simulink model "example1"  (Simulink 10.1)
settings: Solver=ode45  StartTime=0.0  StopTime=15  FixedStep=1e-2  MaxStep=1e-2  RelTol=1e-3  EnableMultiTasking=on
libraries: simulink x3
settings Model: Creator=marcelo  LastModifiedBy=maxwe
settings SolverCC: ZeroCrossAlgorithm=Non-adaptive
settings DataIOCC: SignalLoggingSaveFormat=ModelDataLogs  SaveOutput=off
settings OptimizationCC: ExpressionDepthLimit=2147483647  InitFltsAndDblsToZero=on
settings DebuggingCC: SaveWithParameterizedLinksMsg=none  SignalResolutionControl=TryResolveAllWithWarning  SolverPrmCheckMsg=warning  MultiTaskDSMMsg=warning  MultiTaskCondExecSysMsg=none  FcnCallInpInsideContextMsg=warning  StateNameClashWarn=warning
settings SFSimCC: SimUseLocalCustomCode=on  CustomCodeUndefinedFunction=FilterOut
settings RTWCC: RTWUseLocalCustomCode=on
settings GRTTargetCC: TargetFcnLib=ansi_tfl_tmw.mat
settings ConfigComp: CovExternalEMLEnable=on

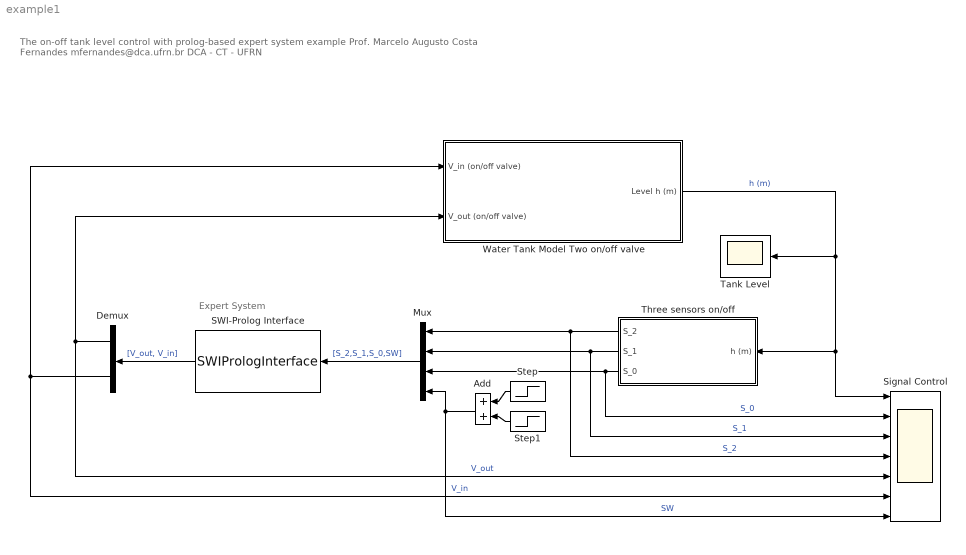
== system example1 ==
  note: Expert System
  note: The on-off tank level control with prolog-based expert system example
      | Prof. Marcelo Augusto Costa Fernandes
      | mfernandes@dca.ufrn.br
      | DCA - CT - UFRN
  Add : Sum
  Demux : Demux  Outputs=2
  Mux : Mux
  SWI-Prolog Interface : S-Function  FunctionName=SWIPrologInterface  Parameters=jplPath, plFile, nIn, plQuery, nOut,0  SFunctionDeploymentMode=off  EnableBusSupport=off  mask(SWI-Prolog (www.swi-prolog.org) Interface){jplPath=E:\Program Files\swipl\lib\jpl.jar, plFile=example1Prolog.pl, nIn=4, nOut=2, plQuery=control(y(2),y(1),u(3),u(2),u(1),u(4))}
      mask prompts: jplPath "Path of the JPL jar-file:"; plFile "Prolog file:"; nIn "Number of the inputs:"; nOut "Number of the outputs:"; plQuery "Prolog query:"
      mask help:
      | SWI-Prolog (www.swi-prolog.org) Interface block.
      |
      | Execute Prolog code (PL file) in the Simulink environment.
      |
      | Use ''u'' as the input variable name and ''y'' as the output variable name.
      |
      | In the case of queries with multiple solutions, this block will only return the first solution found.
      |
      | Prof. Marcelo Augusto Costa Fernandes
      | mfernandes@dca.ufrn.br
      | DCA - CT - UFRN
      mask Help:
      | SWI-Prolog (www.swi-prolog.org) Interface block.
      | 
      | Execute Prolog code (PL file) in the Simulink environment.
      | 
      | Use ''u'' as the input variable name and ''y'' as the output variable name.
      | 
      | In the case of queries with multiple solutions, this block will only return the first solution found.
      | 
      | Prof. Marcelo Augusto Costa Fernandes
      | mfernandes@dca.ufrn.br
      | DCA - CT - UFRN
      mask Display: disp('SWI-Prolog\nInterface')
  Signal Control : Scope  NumInputPorts=7
  Step : Step  SampleTime=0
  Step1 : Step  Time=8  After=-1  SampleTime=0
  Tank Level : Scope
  Three sensors on/off : Subsystem
      mask Display: disp('Three sensors\non/off')
  Water Tank Model Two on/off valve : Subsystem  mask(Water Tank Model){q1=1, h=2, area=1, outletArea=.1}
      mask prompts: q1 "Input flow - q_1 (m^3/s)"; h "Tank height - H (m):"; area "Area - A (m^2):"; outletArea "outlet area (m^2):"
      mask help:
      | Water tank model with two on/off valve: V_in and V_out.
      | V_in is the input valve and V_out is the output valve.
      |
      | Prof. Marcelo Augusto C. Fernandes
      | mfernandes@dca.ufrn.br
      | DCA - CT - UFRN
      mask Display: disp('Water Tank Model\nTwo on/off valve')
  wires:
  Water Tank Model Two on/off valve/1(Level h (m)) -> Signal Control/1, Three sensors on/off/1(h (m)), Tank Level/1  "h (m)"
  Three sensors on/off/3(S_0) -> Signal Control/2, Mux/3  "S_0"
  Three sensors on/off/2(S_1) -> Signal Control/3, Mux/2  "S_1"
  Three sensors on/off/1(S_2) -> Signal Control/4, Mux/1  "S_2"
  Mux/1 -> SWI-Prolog Interface/1  "[S_2,S_1,S_0,SW]"
  SWI-Prolog Interface/1 -> Demux/1  "[V_out, V_in]"
  Demux/1 -> Water Tank Model Two on/off valve/2(V_out (on/off valve)), Signal Control/5  "V_out"
  Demux/2 -> Water Tank Model Two on/off valve/1(V_in (on/off valve)), Signal Control/6  "V_in"
  Step/1 -> Add/1
  Step1/1 -> Add/2
  Add/1 -> Mux/4, Signal Control/7  "SW"

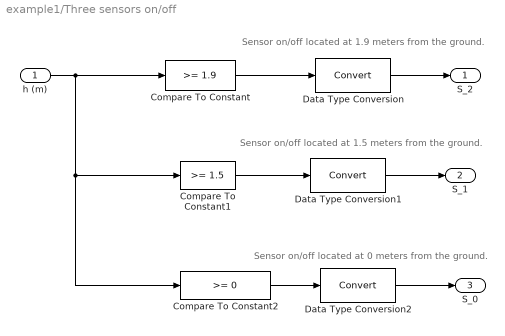
== system example1/Three sensors on/off ==
  note: Sensor on/off located at 0 meters from the ground.
  note: Sensor on/off located at 1.5 meters from the ground.
  note: Sensor on/off located at 1.9 meters from the ground.
  h (m) : Inport
  Compare To Constant : simulink/Logic and Bit Operations/Compare To Constant  relop=>=  const=1.9  OutDataTypeStr=boolean  ZeroCross=off
  Compare To Constant1 : simulink/Logic and Bit Operations/Compare To Constant  relop=>=  const=1.5  OutDataTypeStr=boolean  ZeroCross=off
  Compare To Constant2 : simulink/Logic and Bit Operations/Compare To Constant  relop=>=  const=0  OutDataTypeStr=boolean  ZeroCross=off
  Data Type Conversion : DataTypeConversion
  Data Type Conversion1 : DataTypeConversion
  Data Type Conversion2 : DataTypeConversion
  S_2 : Outport
  S_1 : Outport  Port=2
  S_0 : Outport  Port=3
  wires:
  h (m)/1 -> Compare To Constant/1, Compare To Constant1/1, Compare To Constant2/1
  Compare To Constant/1 -> Data Type Conversion/1
  Compare To Constant2/1 -> Data Type Conversion2/1
  Compare To Constant1/1 -> Data Type Conversion1/1
  Data Type Conversion/1 -> S_2/1
  Data Type Conversion1/1 -> S_1/1
  Data Type Conversion2/1 -> S_0/1

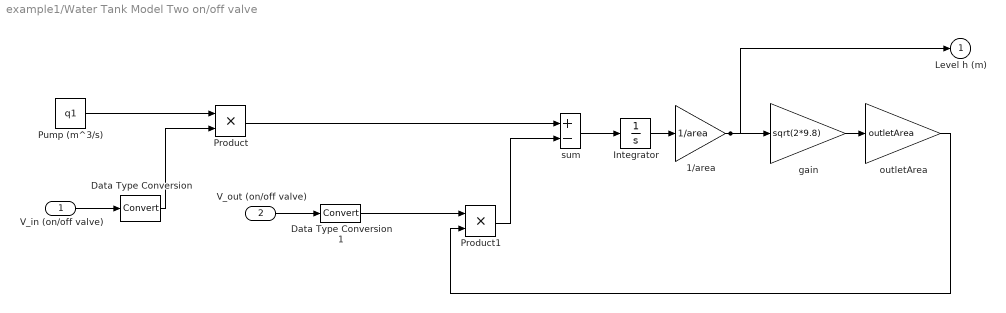
== system example1/Water Tank Model Two on/off valve ==
  V_in (on/off valve) : Inport
  V_out (on/off valve) : Inport  Port=2
  1/area : Gain  Gain=1/area  SaturateOnIntegerOverflow=on  OutDataTypeStr=Inherit: Same as input  ParamDataTypeStr=Inherit: Same as input
  Data Type Conversion : DataTypeConversion
  Data Type Conversion1 : DataTypeConversion
  Integrator : Integrator
  Product : Product  RndMeth=Zero  OutDataTypeStr=Inherit: Same as first input
  Product1 : Product  RndMeth=Zero  OutDataTypeStr=Inherit: Same as first input
  Pump (m^3/s) : Constant  Value=q1
  gain : Gain  Gain=sqrt(2*9.8)  SaturateOnIntegerOverflow=on  OutDataTypeStr=Inherit: Same as input  ParamDataTypeStr=Inherit: Same as input
  outletArea : Gain  Gain=outletArea  SaturateOnIntegerOverflow=on  OutDataTypeStr=Inherit: Same as input  ParamDataTypeStr=Inherit: Same as input
  sum : Sum  Inputs=+-  InputSameDT=on  SaturateOnIntegerOverflow=on  OutDataTypeStr=Inherit: Same as first input
  Level h (m) : Outport  InitialOutput=0
  wires:
  outletArea/1 -> Product1/2
  gain/1 -> outletArea/1
  1/area/1 -> Level h (m)/1, gain/1
  Integrator/1 -> 1/area/1
  Product/1 -> sum/1
  sum/1 -> Integrator/1
  Pump (m^3/s)/1 -> Product/1
  V_in (on/off valve)/1 -> Data Type Conversion/1
  Product1/1 -> sum/2
  Data Type Conversion1/1 -> Product1/1
  V_out (on/off valve)/1 -> Data Type Conversion1/1
  Data Type Conversion/1 -> Product/2
